simulink model "MLP_ideal_case"  (R2024a)
settings: Solver=FixedStepAuto  StartTime=0.0  StopTime=100  FixedStep=1e-3  RelTol=1e-3
settings Model: Creator=erhan  LastModifiedBy=erhan

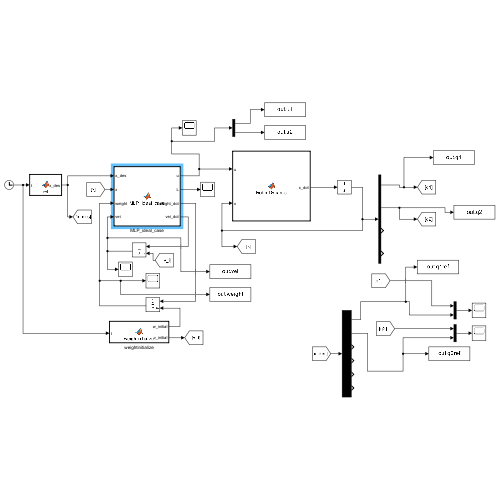
[thumbnail: Simulink's stored preview of the top-level diagram]
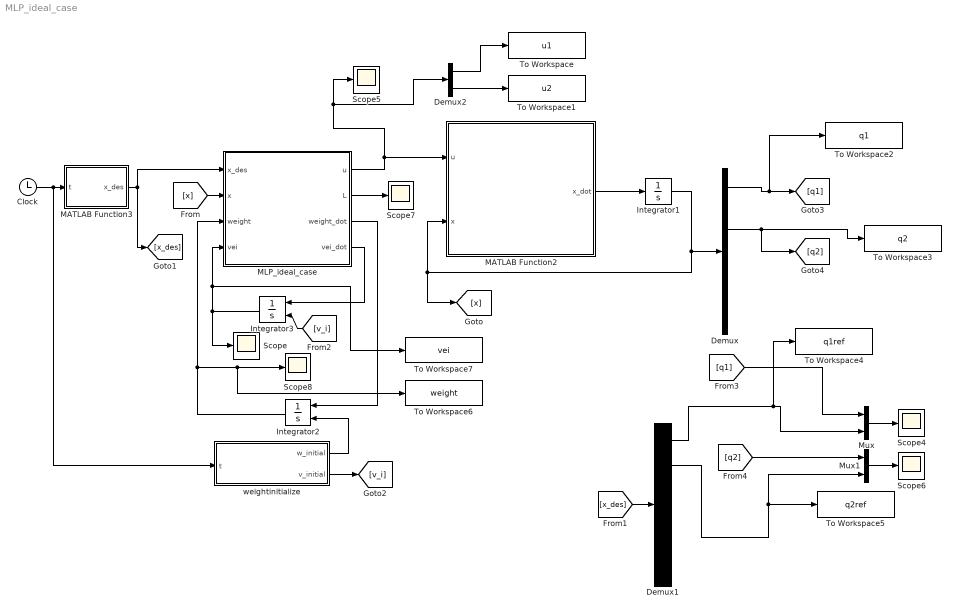
== system MLP_ideal_case ==
  Clock : Clock
  Demux : Demux
  Demux1 : Demux  Outputs=6
  Demux2 : Demux  Outputs=2
  Integrator1 : Integrator  InitialCondition=[0;0;0;0]
  Integrator2 : Integrator  InitialConditionSource=external  InitialCondition=[0;0]
  Integrator3 : Integrator  InitialConditionSource=external  InitialCondition=[0;0]
  MATLAB Function2 : MATLAB Function  TreatAsAtomicUnit=on
  MATLAB Function3 : MATLAB Function  TreatAsAtomicUnit=on
  MLP_ideal_case : MATLAB Function  TreatAsAtomicUnit=on
  Mux : Mux  Inputs=2
  Mux1 : Mux  Inputs=2
  Scope{,4..8} (6 alike) : Scope
  To Workspace : ToWorkspace  VariableName=u1  SaveFormat=Timeseries  SampleTime=-1
  To Workspace1 : ToWorkspace  VariableName=u2  SaveFormat=Timeseries  SampleTime=-1
  To Workspace2 : ToWorkspace  VariableName=q1  SaveFormat=Timeseries  SampleTime=-1
  To Workspace3 : ToWorkspace  VariableName=q2  SaveFormat=Timeseries  SampleTime=-1
  To Workspace4 : ToWorkspace  VariableName=q1ref  SaveFormat=Timeseries  SampleTime=-1
  To Workspace5 : ToWorkspace  VariableName=q2ref  SaveFormat=Timeseries  SampleTime=-1
  To Workspace6 : ToWorkspace  VariableName=weight  SaveFormat=Timeseries  SampleTime=-1
  To Workspace7 : ToWorkspace  VariableName=vei  SaveFormat=Timeseries  SampleTime=-1
  weightinitialize : MATLAB Function  TreatAsAtomicUnit=on
  wires:
  Mux/1 -> Scope4/1
  MLP_ideal_case/1(u) -> MATLAB Function2/1(u), Demux2/1, Scope5/1
  MATLAB Function2/1(x_dot) -> Integrator1/1
  Demux1/1 -> To Workspace4/1, Mux/2
  Demux1/2 -> Mux1/2, To Workspace5/1
  Integrator2/1 -> To Workspace6/1, Scope8/1, MLP_ideal_case/3(weight)
  MLP_ideal_case/2(L) -> Scope7/1
  MATLAB Function3/1(x_des) -> [x_des], MLP_ideal_case/1(x_des)
  Clock/1 -> weightinitialize/1(t), MATLAB Function3/1(t)
  MLP_ideal_case/3(weight_dot) -> Integrator2/1
  Integrator1/1 -> [x], MATLAB Function2/2(x), Demux/1
  Mux1/1 -> Scope6/1
  [x] -> MLP_ideal_case/2(x)
  [x_des] -> Demux1/1
  MLP_ideal_case/4(vei_dot) -> Integrator3/1
  Integrator3/1 -> To Workspace7/1, MLP_ideal_case/4(vei), Scope/1
  weightinitialize/2(v_initial) -> [v_i]
  weightinitialize/1(w_initial) -> Integrator2/2
  [v_i] -> Integrator3/2
  Demux/1 -> To Workspace2/1, [q1]
  Demux/2 -> To Workspace3/1, [q2]
  [q1] -> Mux/1
  [q2] -> Mux1/1
  Demux2/1 -> To Workspace/1
  Demux2/2 -> To Workspace1/1

== matlab function MLP_ideal_case/MATLAB Function2 ==
  data: u input; x_dot output; x input
function x_dot = RobotDynamic(u,x)
% Parametreler
m1=1;
m2=2.3;
L1=1;
L2=1;
g=9.81;

% --- M (Atalet) Matrisi ---
M11 = (L1^2*m1)/3 + L1^2*m2 + (L2^2*m2)/3 + L1*L2*m2*cos(x(2));
M12 = (L2*m2*(2*L2 + 3*L1*cos(x(2))))/6;
M21 = M12;
M22 = (L2^2*m2)/3;

% --- C (Coriolis/Merkezkaç) Vektörü ---
C1 = -(L1*L2*x(3)*m2*sin(x(2))*(2*x(3) + x(4)))/2;
C2 = (L1*L2*x(3)^2*m2*sin(x(2)))/2;

% --- G (Yerçekimi) Vektörü ---
G1 = (g*(L2*m2*cos(x(1) + x(2)) + L1*m1*cos(x(1)) + 2*L1*m2*cos(x(1))))/2;
G2 = (L2*g*m2*cos(x(1) + x(2)))/2;


% N (Nonlinear Terms)
N1 = G1 + C1;
N2 = G2 + C2;

% --- MATRİS TERSİ (Inverse Matrix) HESABI ---
% Determinant
det = M11*M22 - M12*M21;

% HATA BURADAYDI (Düzeltildi)
MI11 = M22/det;
MI12 = -M12/det;
MI21 = -M21/det;  % Eksikti, eklendi.
MI22 = M11/det;   % MI11 yerine MI22 yazildi.

% Giriş Torkları
tau1 = u(1);
tau2 = u(2);

% --- İVMELERİN HESAPLANMASI ---
% Denklem: ddq = inv(M) * (tau - N)
% q(3) -> ddq1
% q(4) -> ddq2

q = zeros(4,1);
q(1) = x(3); % dq1
q(2) = x(4); % dq2

% Matris çarpımı (Manuel):
% ddq1 = MI11*(tau1 - N1) + MI12*(tau2 - N2)
q(3) = MI11*(tau1 - N1) + MI12*(tau2 - N2);

% ddq2 = MI21*(tau1 - N1) + MI22*(tau2 - N2)
q(4) = MI21*(tau1 - N1) + MI22*(tau2 - N2);

x_dot = q;
end

== matlab function MLP_ideal_case/MATLAB Function3 ==
  data: t input; x_des output
function x_des = ref(t)


period = 2;
amp1 = 0.1;
amp2 = 0.1;
fact = 2*pi/period;
sinf = sin(fact*t);
cosf = cos(fact*t);
qd = [amp1*sinf amp2*cosf];
qdp = fact*[amp1*cosf -amp2*sinf];
qdpp = -fact^2*qd;
x_des = [qd qdp qdpp]';

end

== matlab function MLP_ideal_case/MLP_ideal_case ==
  data: x_des input; u output; x input; L output; weight input; weight_dot output; vei input; vei_dot output
function [u,L,weight_dot,vei_dot] = MLP_ideal_case(x_des,x,weight,vei)



Kv = 50*eye(2);
lam = 5*eye(2);
qd = x_des(1:2,1); % angle
qdp = x_des(3:4,1); % velocity
qdpp = x_des(5:6,1); % acceleration
e = qd - [x(1) x(2)]';
ep = qdp - [x(3) x(4)]';
r = ep + lam*e;

%%%%%%%%%% FLNN APP
H=10;
K=2;
I=14;
x_new = [x(1:4)'  x_des(1:6)'  e' ep']; %%%14
v = vei;
w = weight;
sigma_x=zeros(H,1);
sigma_x_dot=zeros(H,1);

% x_m_q = [zeta1'.*1 , zeta1'.*sin(x(1:2)'), zeta1'.*cos(x(1:2)')];
% x_v_m = [zeta2'.*sin(x(1:2)').*x(3:4)', zeta2'.*cos(x(1:2)').*x(3:4)'];
% x_g_q = [cos(x(1:2)'), sin(x(1:2)'), sin(x(1:2)').*cos(x(1:2)'), cos(x(1:2)').*cos(x(1:2)')];
% x_f_qd = [x(3:4)' , sign(x(3:4)')];


% x_m_q = [zeta1'.*1 , zeta1'.*sin(x(1:2)')];
% x_v_m = [zeta2'.*sin(x(1:2)').*x(3:4)'];
% x_g_q = [cos(x(1:2)'), sin(x(1:2)'), cos(x(1:2)').*cos(x(1:2)')];
% x_f_qd = [x(3:4)'];

%%%% output function

for h = 1:1:H
    in_out =0;

    for i = 1:1:length(x_new)
        in_out = in_out + v(i,h)*x_new(1,i);
    end
    sigma_x(h,1) = 1/(1+exp(-in_out));
    sigma_x_dot(h,1) = sigma_x(h,1)*(1*sigma_x(h,1));
end


tau = zeros(K,1);
sigma_x_new = [1;sigma_x];

for k=1:1:K
    cont_in = 0;
    for h =1:1:H+1
        cont_in = cont_in + w(h,k)*sigma_x_new(h,1);
    end
tau(k) = cont_in;
end


%% training algorith


w_dot = zeros(size(w));
v_dot = zeros(size(v));
F = 100;
G=100;

for k=1:1:K
    
    for h =1:1:H+1
        w_dot(h,k)= F*sigma_x_new(h,1)*r(k);
    end
end


for h=1:1:H
    
    for i =1:1:I
        v_dot(i,h)= G*x_new(1,i)*(sigma_x_dot(h,1)*w(h,:)*r);
    end
end

weight_dot = w_dot;
vei_dot = v_dot;
u = tau + Kv*r;
L = 0.5*r'*r;
end

== matlab function MLP_ideal_case/weightinitialize ==
  data: t input; w_initial output; v_initial output
function [w_initial,v_initial] = weightinitialize(t)

H=10;
K=2;
I=14;
v=zeros(I,H);
w=zeros(H+1,K);
w_initial = w;
v_initial = v;

end
